simulink model "VGWEC_Model_FRad"  (R2022a)
settings: Solver=ode3  StartTime=0.0  StopTime=tSim  FixedStep=dt  RelTol=1e-3
undefined symbols (not defined in the file): amp_Wave, AR3, BR3, CR3, DR3, hydroCoeff, hydroVCoeff, I55, test_B, tfRadAR_ROm, tfRadBR_ROm, tfRadCR_ROm, tfRadDR_ROm, theta0, Time_Variant, tRamp, w_Wave, w_WaveIndx, X, Y, Z
libraries: sm_lib x8, nesl_utility x5, simulink x2, cstblocks x1
settings Model: Creator=tdemonte  LastModifiedBy=tdemonte

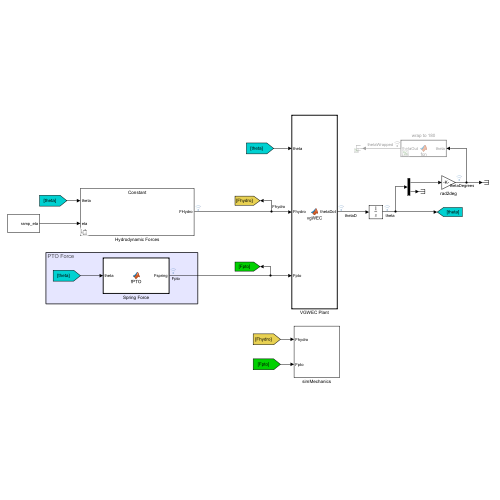
[thumbnail: Simulink's stored preview of the top-level diagram]
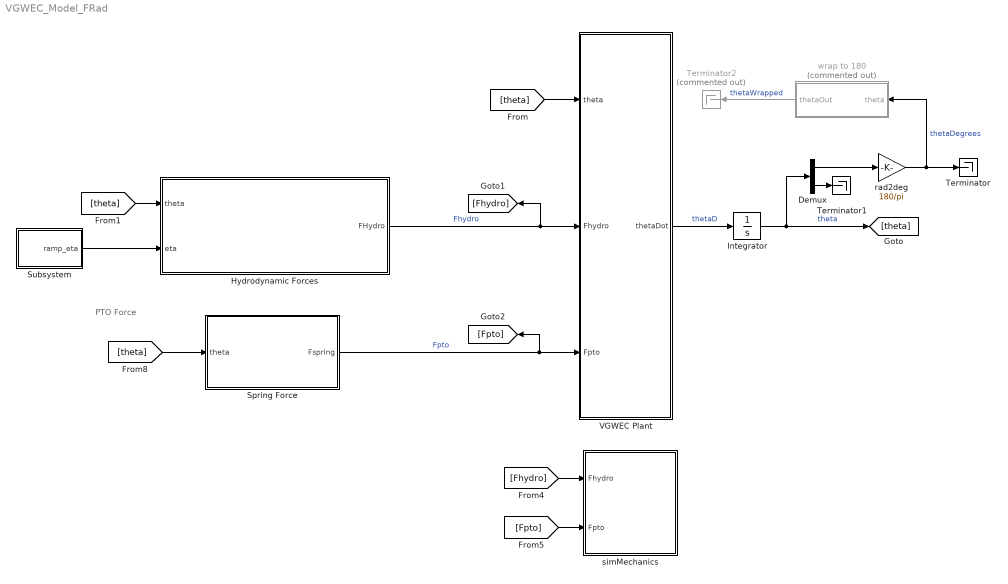
== system VGWEC_Model_FRad ==
  note: PTO Force
  Demux : Demux  Outputs=2
  Hydrodynamic Forces : Subsystem  Variant=on
  Integrator : Integrator  InitialCondition=theta0
  Spring Force : MATLAB Function  TreatAsAtomicUnit=on
  Subsystem : Subsystem
  Terminator : Terminator
  Terminator1 : Terminator
  Terminator2 : Terminator  Commented=on
  VGWEC Plant : MATLAB Function  TreatAsAtomicUnit=on
  rad2deg : Gain  Gain=180/pi
  simMechanics : Subsystem
  wrap to 180 : MATLAB Function  Commented=on  TreatAsAtomicUnit=on
  wires:
  VGWEC Plant/1(thetaDot) -> Integrator/1  "thetaD"
  [theta] -> VGWEC Plant/1(theta)
  rad2deg/1 -> Terminator/1, wrap to 180/1(theta)  "thetaDegrees"
  [theta] -> Spring Force/1(theta)
  Spring Force/1(Fspring) -> [Fpto], VGWEC Plant/3(Fpto)  "Fpto"
  [theta] -> Hydrodynamic Forces/1(theta)
  Hydrodynamic Forces/1(FHydro) -> [Fhydro], VGWEC Plant/2(Fhydro)  "Fhydro"
  [Fhydro] -> simMechanics/1(Fhydro)
  [Fpto] -> simMechanics/2(Fpto)
  Integrator/1 -> Demux/1, [theta]  "theta"
  Subsystem/1(ramp_eta) -> Hydrodynamic Forces/2(eta)
  Demux/1 -> rad2deg/1
  Demux/2 -> Terminator1/1
  wrap to 180/1(thetaOut) -> Terminator2/1  "thetaWrapped"

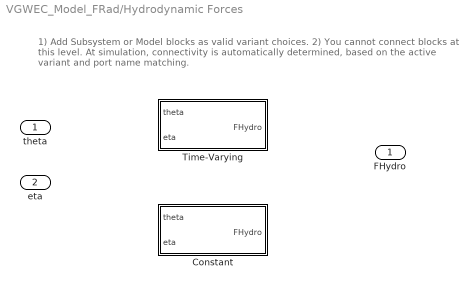
== system VGWEC_Model_FRad/Hydrodynamic Forces ==
  note: 1) Add Subsystem or Model blocks as valid variant choices.
      | 2) You cannot connect blocks at this level. At simulation, connectivity is automatically
      | determined, based on the active variant and port name matching.
  theta : Inport
  eta : Inport  Port=2
  Constant : Subsystem  VariantControl=Time_Variant == 0
  Time-Varying : Subsystem  VariantControl=Time_Variant == 1
  FHydro : Outport

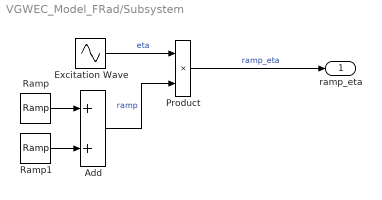
== system VGWEC_Model_FRad/Subsystem ==
  Add : Sum
  Excitation Wave : Sin  Amplitude=amp_Wave  Frequency=w_Wave  SampleTime=0
  Product : Product
  Ramp : simulink/Sources/Ramp  slope=1/tRamp  start=0  InitialOutput=0
  Ramp1 : simulink/Sources/Ramp  slope=-1/tRamp  start=tRamp  InitialOutput=0
  ramp_eta : Outport
  wires:
  Add/1 -> Product/2  "ramp"
  Excitation Wave/1 -> Product/1  "eta"
  Ramp1/1 -> Add/2
  Product/1 -> ramp_eta/1  "ramp_eta"
  Ramp/1 -> Add/1

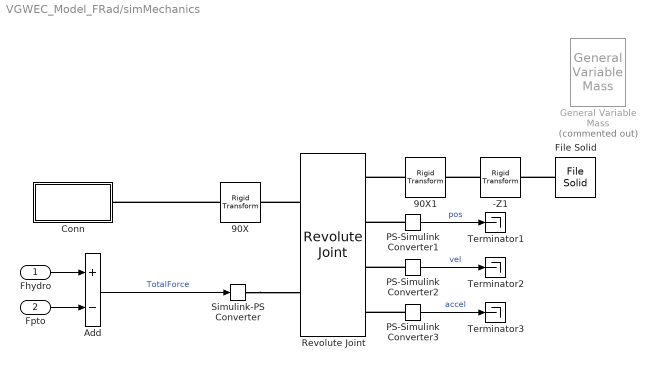
== system VGWEC_Model_FRad/simMechanics ==
  Fhydro : Inport
  Fpto : Inport  Port=2
  -Z1 : sm_lib/Frames and Transforms/Rigid Transform  TranslationMethod=StandardAxis  TranslationStandardOffset=1  TranslationLengthUnit=m  TranslationStandardAxis=+Z  TranslationCartesianOffset=[0 0 ]  TranslationROffset=0  TranslationROffsetUnits=m  TranslationZOffset=0  TranslationZOffsetUnits=m  TranslationThetaOffset=0  TranslationThetaOffsetUnits=deg  RotationMethod=None  RotationAngleUnits=deg  RotationStandardAxis=+X  RotationAngle=90  RotationArbitraryAxis=[0 0 1]  FollAlignAxisA=+X  BaseAlignAxisA=+Y  FollAlignAxisB=+Y  BaseAlignAxisB=+Z  RotationSequenceAxes=FollowerAxes  RotationSequence=XYX  RotationSequenceAngles=[0 0 0]  RotationSequenceAnglesUnits=deg  RotationMatrix=[1 0 0; 0 1 0; 0 0 1]
  90X : sm_lib/Frames and Transforms/Rigid Transform  TranslationMethod=None  TranslationStandardOffset=1  TranslationLengthUnit=m  TranslationStandardAxis=-Y  TranslationCartesianOffset=[0 0 ]  TranslationROffset=0  TranslationROffsetUnits=m  TranslationZOffset=0  TranslationZOffsetUnits=m  TranslationThetaOffset=0  TranslationThetaOffsetUnits=deg  RotationMethod=StandardAxis  RotationAngleUnits=deg  RotationStandardAxis=+X  RotationAngle=90  RotationArbitraryAxis=[0 0 1]  FollAlignAxisA=+X  BaseAlignAxisA=+Y  FollAlignAxisB=+Y  BaseAlignAxisB=+Z  RotationSequenceAxes=FollowerAxes  RotationSequence=XYX  RotationSequenceAngles=[0 0 0]  RotationSequenceAnglesUnits=deg  RotationMatrix=[1 0 0; 0 1 0; 0 0 1]
  90X1 : sm_lib/Frames and Transforms/Rigid Transform  TranslationMethod=None  TranslationStandardOffset=0  TranslationLengthUnit=m  TranslationStandardAxis=+Z  TranslationCartesianOffset=[0 -1 0]  TranslationROffset=0  TranslationROffsetUnits=m  TranslationZOffset=0  TranslationZOffsetUnits=m  TranslationThetaOffset=0  TranslationThetaOffsetUnits=deg  RotationMethod=StandardAxis  RotationAngleUnits=deg  RotationStandardAxis=-X  RotationAngle=90  RotationArbitraryAxis=[0 0 1]  FollAlignAxisA=+X  BaseAlignAxisA=+Y  FollAlignAxisB=+Y  BaseAlignAxisB=+Z  RotationSequenceAxes=FollowerAxes  RotationSequence=XYX  RotationSequenceAngles=[0 0 0]  RotationSequenceAnglesUnits=deg  RotationMatrix=[1 0 0; 0 1 0; 0 0 1]
  Add : Sum  Inputs=+-
  Conn : Subsystem
  File Solid : sm_lib/Body Elements/File Solid  ExtGeomFileName=C:\Users\tdemonte\OneDrive - NREL\VGWEC\Full Flap Data\flap0deg.STL  UnitType=Custom  ExtGeomFileUnits=mm  StepReaderType=HEX  ExportConvexHullGeometry=off  InertiaType=Custom  Mass=I55  MassUnits=kg  CenterOfMass=[0 0 -1]  CenterOfMassUnits=m  MomentsOfInertia=[1 hydroVCoeff.IA(hydroCoeff.singleThetaIndex) + hydroCoeff.IQ 1]  MomentsOfInertiaUnits=kg*m^2  ProductsOfInertia=[0 0 0]  ProductsOfInertiaUnits=kg*m^2  BasedOnType=Mass  Density=1000  DensityUnits=kg/m^3  DoExposeReferenceFrame=on  SerializedFrames=<Frames/>  GraphicType=FromGeometry  MarkerShape=Sphere  MarkerSize=10  GraphicVisPropType=SimpleVisualProperties  GraphicDiffuseColor=[0.5 0.5 0.5]  GraphicSpecularColor=[0.5 0.5 0.5 1.0]  GraphicAmbientColor=[0.15 0.15 0.15 1.0]  GraphicEmissiveColor=[0.0 0.0 0.0 1.0]  GraphicShininess=75  GraphicOpacity=0.5
  General Variable Mass : sm_lib/Body Elements/Variable Mass/General Variable Mass  Commented=on  VariableInertiaType=Custom  MassType=TimeVarying  Mass=1  MassUnits=kg  CenterOfMassType=Constant  CenterOfMass=[0 0 0]  CenterOfMassUnits=m  InertiaMatrixType=Constant  MomentsOfInertia=[1 1 1]  MomentsOfInertiaUnits=kg*m^2  ProductsOfInertia=[0 0 0]  ProductsOfInertiaUnits=kg*m^2  GraphicType=InertiaEllipsoid  MarkerShape=Sphere  MarkerSize=10  GraphicVisPropType=SimpleVisualProperties  GraphicDiffuseColor=[0.5 0.5 0.5]  GraphicSpecularColor=[0.5 0.5 0.5 1.0]  GraphicAmbientColor=[0.15 0.15 0.15 1.0]  GraphicEmissiveColor=[0.0 0.0 0.0 1.0]  GraphicShininess=75  GraphicOpacity=1.0
      settings: SourceProductBaseCode=MS
  PS-Simulink Converter1 : nesl_utility/PS-Simulink Converter  PhysicalDomain=network_engine_domain  SubClassName=ps_output  LeftPortType=input  RightPortType=output  PseudoPeriodic=off  Frequencies=[]  VectorFormat=inherit  Unit=inherit  AffineConversion=off
      settings: SourceProductBaseCode=SS,PW,VE
  PS-Simulink Converter2 : nesl_utility/PS-Simulink Converter  PhysicalDomain=network_engine_domain  SubClassName=ps_output  LeftPortType=input  RightPortType=output  PseudoPeriodic=off  Frequencies=[]  VectorFormat=inherit  Unit=inherit  AffineConversion=off
      settings: SourceProductBaseCode=SS,PW,VE
  PS-Simulink Converter3 : nesl_utility/PS-Simulink Converter  PhysicalDomain=network_engine_domain  SubClassName=ps_output  LeftPortType=input  RightPortType=output  PseudoPeriodic=off  Frequencies=[]  VectorFormat=inherit  Unit=inherit  AffineConversion=off
      settings: SourceProductBaseCode=SS,PW,VE
  Revolute Joint : sm_lib/Joints/Revolute Joint  JointMode=Normal  SenseConstraintForce=off  SenseConstraintForceX=off  SenseConstraintForceY=off  SenseConstraintForceZ=off  SenseConstraintTorque=off  SenseConstraintTorqueX=off  SenseConstraintTorqueY=off  SenseConstraintTorqueZ=off  SenseTotalForce=off  SenseTotalForceX=off  SenseTotalForceY=off  SenseTotalForceZ=off  SenseTotalTorque=off  SenseTotalTorqueX=off  SenseTotalTorqueY=off  SenseTotalTorqueZ=off  CompositeWrenchDir=FollowerOnBase  CompositeWrenchFrame=BaseFrame  EquilibriumPosition=0  EquilibriumPositionUnits=deg  SpringStiffness=0  SpringStiffnessUnits=N*m/deg  DampingCoefficient=0  DampingCoefficientUnits=N*m/(deg/s)  TorqueActuationMode=InputTorque  MotionActuationMode=ComputedMotion  SensePosition=on  SenseVelocity=on  SenseAcceleration=on  SenseTorqueForce=off  SenseLowerLimitTorqueForce=off  SenseUpperLimitTorqueForce=off  LowerLimitSpecify=off  LowerLimitBound=-90  LowerLimitBoundUnits=deg  LowerLimitStiffness=1e4  LowerLimitStiffnessUnits=N*m/deg  LowerLimitDamping=10  LowerLimitDampingUnits=N*m/(deg/s)  LowerLimitTransitionRegionWidth=0.1  LowerLimitTransitionRegionWidthUnits=deg  UpperLimitSpecify=off  UpperLimitBound=90  UpperLimitBoundUnits=deg  UpperLimitStiffness=1e4  UpperLimitStiffnessUnits=N*m/deg  UpperLimitDamping=10  UpperLimitDampingUnits=N*m/(deg/s)  UpperLimitTransitionRegionWidth=0.1  UpperLimitTransitionRegionWidthUnits=deg  PositionTargetSpecify=off  PositionTargetPriority=High  PositionTargetValue=0  PositionTargetValueUnits=deg  VelocityTargetSpecify=off  VelocityTargetPriority=High  VelocityTargetValue=0  VelocityTargetValueUnits=deg/s
  Simulink-PS Converter : nesl_utility/Simulink-PS Converter  PhysicalDomain=network_engine_domain  SubClassName=ps_input  LeftPortType=input  RightPortType=output  PseudoPeriodic=off  Frequencies=[]  NoiseDistribution=none  NoiseParameters=[]  Unit=1  AffineConversion=off  FilteringAndDerivatives=provide  SimscapeFilterOrder=1  InputFilterTimeConstant=0.001  UdotUserProvided=0
      settings: SourceProductBaseCode=SS,PW,VE
  Terminator1 : Terminator
  Terminator2 : Terminator
  Terminator3 : Terminator
  wires:
  Add/1 -> Simulink-PS Converter/1  "TotalForce"
  PS-Simulink Converter3/1 -> Terminator3/1  "accel"
  PS-Simulink Converter2/1 -> Terminator2/1  "vel"
  PS-Simulink Converter1/1 -> Terminator1/1  "pos"
  Fhydro/1 -> Add/1
  Fpto/1 -> Add/2
  connections:
  PS-Simulink Converter3/LConn1 -- Revolute Joint/RConn4
  File Solid/RConn1 -- -Z1/RConn1
  PS-Simulink Converter2/LConn1 -- Revolute Joint/RConn3
  PS-Simulink Converter1/LConn1 -- Revolute Joint/RConn2
  Simulink-PS Converter/RConn1 -- Revolute Joint/LConn2
  Revolute Joint/LConn1 -- 90X/RConn1
  90X1/LConn1 -- Revolute Joint/RConn1
  90X/LConn1 -- Conn/RConn1
  -Z1/LConn1 -- 90X1/RConn1

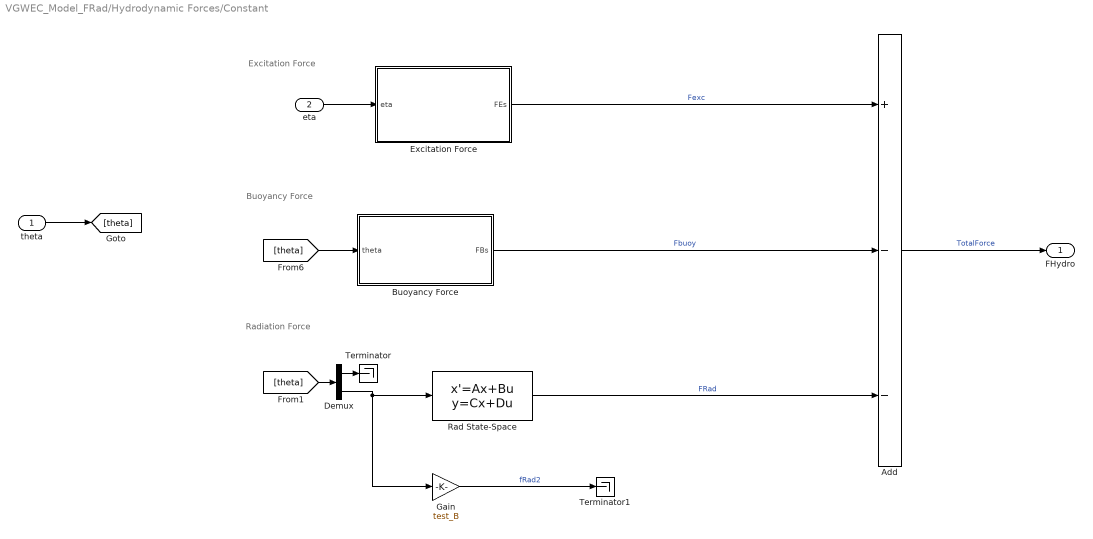
== system VGWEC_Model_FRad/Hydrodynamic Forces/Constant ==
  note: Excitation Force
  note: Radiation Force
  note: Buoyancy Force
  theta : Inport
  eta : Inport  Port=2
  Add : Sum  Inputs=+--
  Buoyancy Force : MATLAB Function  TreatAsAtomicUnit=on
  Demux : Demux  Outputs=2
  "Excitation Force " : MATLAB Function  TreatAsAtomicUnit=on
  Gain : Gain  Gain=test_B
  Rad State-Space : StateSpace  A=AR3  B=BR3  C=CR3  D=DR3  InitialCondition=0
  Terminator : Terminator
  Terminator1 : Terminator
  FHydro : Outport
  wires:
  "Excitation Force "/1(FEs) -> Add/1  "Fexc"
  Demux/2 -> Gain/1, Rad State-Space/1
  Buoyancy Force/1(FBs) -> Add/2  "Fbuoy"
  eta/1 -> "Excitation Force "/1(eta)
  theta/1 -> [theta]
  [theta] -> Buoyancy Force/1(theta)
  Rad State-Space/1 -> Add/3  "FRad"
  Demux/1 -> Terminator/1
  [theta] -> Demux/1
  Add/1 -> FHydro/1  "TotalForce"
  Gain/1 -> Terminator1/1  "fRad2"

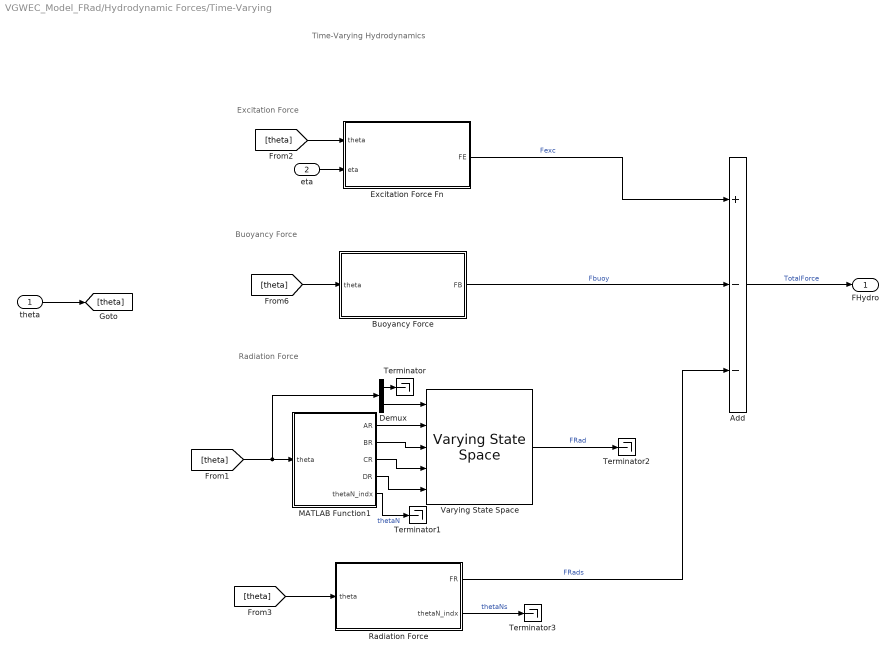
== system VGWEC_Model_FRad/Hydrodynamic Forces/Time-Varying ==
  note: Time-Varying Hydrodynamics
  note: Excitation Force
  note: Radiation Force
  note: Buoyancy Force
  theta : Inport
  eta : Inport  Port=2
  Add : Sum  Inputs=+--
  Buoyancy Force : MATLAB Function  TreatAsAtomicUnit=on
  Demux : Demux  Outputs=2
  Excitation Force Fn : MATLAB Function  TreatAsAtomicUnit=on
  MATLAB Function1 : MATLAB Function  TreatAsAtomicUnit=on
  Radiation Force : MATLAB Function  TreatAsAtomicUnit=on
  Terminator{,1..3} (4 alike) : Terminator
  Varying State Space : cstblocks/Linear Parameter Varying/Varying State Space  x0=0  xNames=''  OutputX=off  OutputDX=off
  FHydro : Outport
  wires:
  [theta] -> Buoyancy Force/1(theta)
  [theta] -> Excitation Force Fn/1(theta)
  Varying State Space/1 -> Terminator2/1  "FRad"
  MATLAB Function1/4(DR) -> Varying State Space/5
  MATLAB Function1/3(CR) -> Varying State Space/4
  MATLAB Function1/2(BR) -> Varying State Space/3
  MATLAB Function1/1(AR) -> Varying State Space/2
  [theta] -> Demux/1, MATLAB Function1/1(theta)
  theta/1 -> [theta]
  Demux/2 -> Varying State Space/1
  Demux/1 -> Terminator/1
  Add/1 -> FHydro/1  "TotalForce"
  Excitation Force Fn/1(FE) -> Add/1  "Fexc"
  Buoyancy Force/1(FB) -> Add/2  "Fbuoy"
  eta/1 -> Excitation Force Fn/2(eta)
  [theta] -> Radiation Force/1(theta)
  Radiation Force/1(FR) -> Add/3  "FRads"
  MATLAB Function1/5(thetaN_indx) -> Terminator1/1  "thetaN"
  Radiation Force/2(thetaN_indx) -> Terminator3/1  "thetaNs"

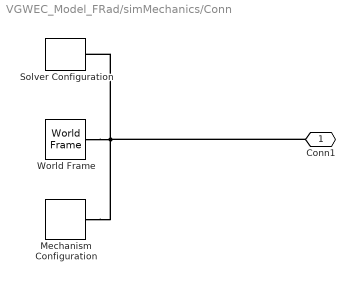
== system VGWEC_Model_FRad/simMechanics/Conn ==
  Mechanism Configuration : sm_lib/Utilities/Mechanism Configuration  UniformGravity=Constant  GravityVector=[0 0 -9.80665]  GravityUnits=m/s^2  LinearizationDelta=0.001  JointModeTransitionNonlinearIterations=2
  Solver Configuration : nesl_utility/Solver Configuration  PhysicalDomain=network_engine_domain  SubClassName=solver  LeftPortType=input  RightPortType=generic  Tones=[]  Harmonics=[]  SimulateNoise=off  Profile=off  UseLocalSampling=off  EnableSwitchedLinearOptims=on  FrequencyDomain=off  UseCCode=off  RelTol=0.001  AbsTol=1e-06  MinStep=1e-09  ToWorkspace=off  RevertToSquareIcSolve=off  NumHomotopyIterations=100  PhasorMode=off  PhasorModeNumHarmonics=1  IndexReductionMethod=DerivativeReplacement  DoDC=off  ResidualTolerance=1e-09  UseLocalSolver=off  LocalSolverChoice=NE_BACKWARD_EULER_ADVANCER  LocalSolverSampleTime=0.001  DoFixedCost=off  MaxNonlinIter=3  MaxModeIter=2  ComputeImpulses=off  ImpulseIterations=2  LinearAlgebra=Sparse  LinearAlgebraNumThread=0  EquationFormulation=NE_TIME_EF  DelaysMemoryBudget=1024  AutomaticFiltering=on  FilteringTimeConstant=0.001  PartitionStorageMethod=AS_NEEDED  PartitionMemoryBudget=1024  PartitionMethod=FAST
      settings: SourceProductBaseCode=SS,PW,VE
  World Frame : sm_lib/Frames and Transforms/World Frame
  Conn1 : PMIOPort  Side=Right
  connections:
  World Frame/RConn1 -- Solver Configuration/RConn1 -- Mechanism Configuration/RConn1 -- Conn1/RConn1

== matlab function VGWEC_Model_FRad/Hydrodynamic Forces/Constant/Excitation Force  ==
  data: eta input size=1; hydroCoeff parameter; hydroVCoeff parameter; w_Wave parameter; FEs output size=1
function  FEs = fE(eta,hydroCoeff, hydroVCoeff, w_Wave)


%% Calculate the Excitation Force for a Constant theta
w  = find(hydroCoeff.w > w_Wave,1)-1;
KE = hydroVCoeff.KE(w, hydroCoeff.singleThetaIndex); % Excitation Force Kernel

FEs = 0; 
FEs(1) = eta*KE;

== matlab function VGWEC_Model_FRad/wrap to 180 ==
  data: theta input; thetaOut output
function thetaOut = fcn(theta)

thetaOut = 0; 
thetaOut(1) = wrapTo180(theta);

thetaOut = theta;

== matlab function VGWEC_Model_FRad/VGWEC Plant ==
  data: theta input size=2; thetaDot output size=[1 2]; Fhydro input size=1; hydroVCoeff parameter; hydroCoeff parameter; Fpto input; Time_Variant parameter
function thetaDot = vgWEC(theta, Fhydro, hydroVCoeff, hydroCoeff, Fpto, Time_Variant)

% Declare the plant as an extrinsic function
%coder.extrinsic('vgWecPlant');

thetaDot = vgWecPlant(theta, hydroCoeff, hydroVCoeff, Fhydro, Fpto, Time_Variant);

%% Wrap the angle to be +- Pi 

% thetaDot = wrapToPi(thetaDot);

== matlab function VGWEC_Model_FRad/Hydrodynamic Forces/Time-Varying/Radiation Force ==
  data: theta input size=[1 2]; FR output double size=1; hydroCoeff parameter; hydroVCoeff parameter; w_WaveIndx parameter; thetaN_indx output
function [FR, thetaN_indx] = fRad(theta,hydroCoeff, hydroVCoeff,w_WaveIndx)

% States: 
theta1  = theta(1); % (1) theta:  pitch angle response
theta2  = theta(2); % (2) thetaD: pitch angle velocity

% Find the index for the discretized theta 

theta1N = wrapToPi(theta1); 

if abs(rad2deg(theta1N)) >= 95 
    theta1N = pi - abs(theta1N);
end 


thetaN = find(deg2rad(hydroCoeff.theta) > abs(theta1N),1); 

thetaN_indx = 0; 
thetaN_indx = thetaN(1);

b  = hydroVCoeff.KR(w_WaveIndx,thetaN); % Radiation Damping Coefficient  

FR = 0; 
FR(1) = b*theta2; % Buoyancy Force for Time-Varying Hydrodynamics (N)

== matlab function VGWEC_Model_FRad/Hydrodynamic Forces/Time-Varying/Buoyancy Force ==
  data: theta input size=[1 2]; FB output double size=1; hydroCoeff parameter; hydroVCoeff parameter
function FB = fBuoy(theta,hydroCoeff, hydroVCoeff)

% States: 
theta1  = theta(1); % (1) theta:  pitch angle response
% theta2  = theta(2); % (2) thetaD: pitch angle velocity

% Find the index for the discretized theta 

theta1N = wrapToPi(theta1); 

if abs(rad2deg(theta1N)) >= 95 
    theta1N = pi - abs(theta1N);
end 


thetaN = find(deg2rad(hydroCoeff.theta) > abs(theta1N),1); 

c  = hydroVCoeff.c(thetaN); % Hydrostatic restoring coefficient. (t) 
FB = 0; 
FB(1) = c*theta1; % Buoyancy Force for Time-Varying Hydrodynamics (N)

== matlab function VGWEC_Model_FRad/Hydrodynamic Forces/Time-Varying/Excitation Force Fn ==
  data: theta input size=[1 2]; FE output double size=1; eta input size=1; hydroCoeff parameter; hydroVCoeff parameter; w_Wave parameter
function FE= fE(theta,eta,hydroCoeff, hydroVCoeff, w_Wave)

% % Declare the excitation force function as an extrinsic function
% %coder.extrinsic('fExc');
% 
% FE = fExc(theta, eta, w_Wave,hydroVCoeff,hydroCoeff);
% 
% function FE = fExc(theta, eta, w_Wave,hydroVCoeff,hydroCoeff)
% This function generates the linear excitation force

% Inputs: 
% theta0      = current states condition
% eta         = wave excitation (m)
% w_Wave      = wave excitation angular frequency 'Omega' (rad/s)
% hydroCoeff  = time-invariable hydrodynamic coefficients
% hydrovCoeff = time-variable hydrodynamic coefficients


% Outputs: 
% FE    = excitation force (N) 
theta1 = theta(1); 

% Find the index for the discretized theta 
% if abs(rad2deg(theta1)) > 180 && abs(rad2deg(theta1)) < 360
%     theta1 = 360 - abs(rad2deg(theta1));
%     theta1 = deg2rad(theta1);
% end 
% 
% if abs(rad2deg(theta1)) >= 95 && abs(rad2deg(theta1)) < 180
%     theta1 = 180 - abs(rad2deg(theta1));
%     theta1 = deg2rad(theta1);
% end 

theta1N = wrapToPi(theta1); 

if abs(rad2deg(theta1N)) >= 95 
    theta1N = pi - abs(theta1N); 
end 

theta1Ndeg = rad2deg(theta1N);

thetaN = find(deg2rad(hydroCoeff.theta) > abs(theta1N),1); 


% Find the index for the wave excitation frequency 
w  = find(hydroCoeff.w > w_Wave,1)-1;

% thetaN = 1; 
% w  = 13; 

KE = hydroVCoeff.KE(w, thetaN); % Added mass moment of inertia at inf. freq. (t)

FE = zeros(1,1); 
FE(1) = eta*KE;

== matlab function VGWEC_Model_FRad/Hydrodynamic Forces/Constant/Buoyancy Force ==
  data: theta input size=[1 2]; FBs output double size=1; hydroCoeff parameter; hydroVCoeff parameter
function FBs = fBuoy(theta,hydroCoeff, hydroVCoeff)

% States: 
theta1  = theta(1); % (1) theta:  pitch angle response
% theta2  = theta(2); % (2) thetaD: pitch angle velocity

% Find the index for the discretized theta 
% if abs(rad2deg(theta1)) > 100
%     theta1 = 180 - abs(rad2deg(theta1));
%     theta1 = deg2rad(theta1);
% end 

%% Constant Theta
cs  = hydroVCoeff.c(hydroCoeff.singleThetaIndex); % Hydrostatic restoring coefficient. (t) 
FBs = 0; 
FBs(1) = cs*theta1;

== matlab function VGWEC_Model_FRad/Hydrodynamic Forces/Time-Varying/MATLAB Function1 ==
  data: theta input; AR output size=[6 6]; BR output size=[6 1]; CR output size=[1 6]; DR output size=1; hydroCoeff parameter; tfRadAR_ROm parameter; tfRadBR_ROm parameter; tfRadCR_ROm parameter; tfRadDR_ROm parameter; thetaN_indx output size=1
function [AR, BR, CR, DR, thetaN_indx] = RadTFCoeffs(theta,hydroCoeff, tfRadAR_ROm, tfRadBR_ROm, tfRadCR_ROm, tfRadDR_ROm)
% This function extracts the coefficients of the Radiation Transfer
% Function based on previously fitted data between discretized thetas. 

% Inputs: 
% theta0      = current states condition
% hydrovCoeff = time-variable hydrodynamic coefficients
% thetaN      = pitch angle index

% Outputs: 
% bR    = radiation force (N) 

theta1 = theta(1); 
% Find the index for the discretized theta 
theta1N = wrapToPi(theta1); 

if abs(rad2deg(theta1N)) >= 95 
    theta1N = pi - abs(theta1N);
end 

 
thetaN = find(deg2rad(hydroCoeff.theta) > abs(theta1N),1); 

% % Get transfer function coefficients depending on the discretized angle. 
AR       = zeros(6,6); 
BR       = zeros(6,1); 
CR       = zeros(1,6); 
DR       = 0; 

thetaN_indx = 0; 
thetaN_indx = thetaN(1);

AR(:,:)       = tfRadAR_ROm(:,(thetaN_indx-1)*6+1:(thetaN_indx*6)); % A Matrix Coefficients

BR(:,1)       = tfRadBR_ROm(:,thetaN_indx); % A Matrix Coefficients
CR(1,:)       = tfRadCR_ROm(1,(thetaN_indx-1)*6+1:(thetaN_indx*6)); % A Matrix Coefficients
DR(1)         = tfRadDR_ROm(thetaN_indx); % A Matrix Coefficients

== matlab function VGWEC_Model_FRad/Spring Force ==
  data: theta input size=2; Fspring output size=1; hydroCoeff parameter
function Fspring = fPTO(theta,hydroCoeff)

% This function represents the plant of a variable geometry wave energy
% converter. The model here is derived by Mcabe 2006. 

% Inputs: 
% theta      = initial state conditions
% hydroCoeff  = time-invariable hydrodynamic coefficients

% Outputs: 
% Fspring   = PTO spring force

% States: 
theta1  = theta(1); % (1) theta:  pitch angle response
% theta2  = theta(2); % (2) thetaD: pitch angle velocity

% Spring Force to keep the flap from rotating
K       = hydroCoeff.Kspring;  % Spring Constant
Fspring = K * theta1; 

end
